simulink model "truck_mpc_8dof_2020a"  (R2020a)
settings: Solver=FixedStepAuto  StartTime=0.0  StopTime=40  FixedStep=0.001  RelTol=1e-3
libraries: neural x31, simulink x2, Solver_SF x1
(part 2 of 2)

== system truck_mpc_8dof_2020a/Feed-Forward Neural Network/Layer 4/Delays 1 ==
  "p{4}" : Inport  PortDimensions=6  SampleTime=0.0005
      mask Display: e = 0.06;c1 = [120 230 180]/255;c2 = ([120 230 180]+0)/(256+128);c3 = ([120 230 180]+128)/(256+128);patch([0 1 1 0],[0 0 1 1],c1);patch([0 1 1 1-e 1-e 0+e],[0 0 1 1-e 0+e 0+e],c2);patch([0 0 1 1-e 0+e 0+e],[0 1 1 1-e 1-e 0+e],c3);plot([0 1 1 0 0],[0 0 1 1 0]);
  mux : Mux  Inputs=1
      mask Display: e = 0.06;c1 = [120 150 230]/255;c2 = ([120 150 230]+0)/383;c3 = ([120 150 230]+128)/383;patch([0 1 1 0],[0 0 1 1],c1);patch([0 1 1 1-e 1-e 0+e],[0 0 1 1-e 0+e 0+e],c2);patch([0 0 1 1-e 0+e 0+e],[0 1 1 1-e 1-e 0+e],c3);plot([0 1 1 0 0],[0 0 1 1 0]);disp('Mux')
  "pd{4,3}" : Outport
      mask Display: e = 0.06;c1 = [120 230 180]/255;c2 = ([120 230 180]+0)/(256+128);c3 = ([120 230 180]+128)/(256+128);patch([0 1 1 0],[0 0 1 1],c1);patch([0 1 1 1-e 1-e 0+e],[0 0 1 1-e 0+e 0+e],c2);patch([0 0 1 1-e 0+e 0+e],[0 1 1 1-e 1-e 0+e],c3);plot([0 1 1 0 0],[0 0 1 1 0]);
  wires:
  "p{4}"/1 -> mux/1
  mux/1 -> "pd{4,3}"/1

== system truck_mpc_8dof_2020a/Feed-Forward Neural Network/Layer 4/LW{4,3} ==
  "ad{4,3}" : Inport  PortDimensions=6  SampleTime=0.0005
      mask Display: e = 0.06;c1 = [120 230 180]/255;c2 = ([120 230 180]+0)/(256+128);c3 = ([120 230 180]+128)/(256+128);patch([0 1 1 0],[0 0 1 1],c1);patch([0 1 1 1-e 1-e 0+e],[0 0 1 1-e 0+e 0+e],c2);patch([0 0 1 1-e 0+e 0+e],[0 1 1 1-e 1-e 0+e],c3);plot([0 1 1 0 0],[0 0 1 1 0]);
  "IW{4,3}(1,:)'" : Constant  Value=[1.0365086789271795719713509242865256965160369873046875;-0.07770699028544313102795371150932624004781246185302734375;-0.9449999401189803638345665603992529213428497314453125;0.1511782678576858440777641590102575719356536865234375;0.25449790728671828343721017517964355647563934326171875;-1.6818672952565700828841954717063345015048980712890625]
      mask Display: e = 0.06;c1 = [120 150 230]/255;c2 = ([120 150 230]+0)/383;c3 = ([120 150 230]+128)/383;patch([0 1 1 0],[0 0 1 1],c1);patch([0 1 1 1-e 1-e 0+e],[0 0 1 1-e 0+e 0+e],c2);patch([0 0 1 1-e 0+e 0+e],[0 1 1 1-e 1-e 0+e],c3);plot([0 1 1 0 0],[0 0 1 1 0]);disp('weights');
  Mux : Mux  Inputs=1
      mask Display: e = 0.06;c1 = [120 150 230]/255;c2 = ([120 150 230]+0)/383;c3 = ([120 150 230]+128)/383;patch([0 1 1 0],[0 0 1 1],c1);patch([0 1 1 1-e 1-e 0+e],[0 0 1 1-e 0+e 0+e],c2);patch([0 0 1 1-e 0+e 0+e],[0 1 1 1-e 1-e 0+e],c3);plot([0 1 1 0 0],[0 0 1 1 0]);disp('Mux');
  dotprod1 : neural/Weight Functions/dotprod
  "lz{4,3}" : Outport
      mask Display: e = 0.06;c1 = [120 230 180]/255;c2 = ([120 230 180]+0)/(256+128);c3 = ([120 230 180]+128)/(256+128);patch([0 1 1 0],[0 0 1 1],c1);patch([0 1 1 1-e 1-e 0+e],[0 0 1 1-e 0+e 0+e],c2);patch([0 0 1 1-e 0+e 0+e],[0 1 1 1-e 1-e 0+e],c3);plot([0 1 1 0 0],[0 0 1 1 0]);
  wires:
  "IW{4,3}(1,:)'"/1 -> dotprod1/1
  "ad{4,3}"/1 -> dotprod1/2
  dotprod1/1 -> Mux/1
  Mux/1 -> "lz{4,3}"/1

== matlab function truck_mpc_8dof_2020a/Speed PID controller/MATLAB Function1 ==
  data: u input; th output; b output
function [th, b]= fcn(u)

if u >= 0
    th=u;
    b=0;
elseif u<0
    th=0;
    b=u;
else
    th = 0;
    b = 0;
end

== matlab function truck_mpc_8dof_2020a/MPC Controller/MPC controller ==
  data: Xo input; steer output; Yo input; Yaw input; Yr input; V input; Vy input; Yaw_rate input; Yawr input
function steer = fcn(Xo, Yo, Yaw, Yr, V, Vy, Yaw_rate, Yawr)
x_k = [Yo-Yr;
       Yaw - Yawr;
       0;
       0]; %后两维可以编写一个误差获取的模块加在前面
N = 100;
%定义系统矩阵
q=[10,10,1,1];
Q = diag(q);
R = 1;
T = 0.001;

kf=140000;
km=120000;
kr=120000;
m=61000;
Iz=23665;
a=2.2;
b=2;
c=3.9;

if V <= 0.5
    V = 0.5;
end

tildeA = [1 V*T           T                              0                           ;
          0 1             0                              T                           ;
          0 0             1-T*(kf+km+kr)/(m*V)           -T*(a*kf-b*km-c*kr)/(m*V)-V*T    ;
          0 0             -T*(a*kf-b*km-c*kr)/(Iz*V)      1-T*(a*a*kf+b*b*km+c*c*kr)/(Iz*V)];

tildeB = [0;
          0;
          T*kf/m;
          T*a*kf/Iz];


n = size(tildeA,1);
p = size(tildeB,2);

Psi = zeros(N*n, n);
Theta = zeros(N*n,N*p);
tmp=eye(n);


for i = 1:N
    rows = (i-1)*n+(1:n);
    if i == 1
        Theta(rows, 1:p) = tmp*tildeB;
    else
        Theta(rows, :) = [tmp*tildeB, Theta(rows-n, 1:end-p)];
    end
    tmp = tildeA*tmp;
    Psi(rows,:) = tmp;
end

Q_bar = kron(eye(N),Q);
R_bar = kron(eye(N),R);

E = Theta'*Q_bar*Psi;
H = Theta'*Q_bar*Theta + R_bar;
error = Psi*x_k;
% print(size(error))
U_k = zeros(N*p, 1);
U_k = -H^-1*E*x_k;

steer = U_k(1:p,1);%1:p



% function steer = fcn(Xo, Yo ,Yaw, Yr, V, deltar)
% x_k = [Yo-Yr;
%         Yaw;
%         0];
% N = 100;
% %定义系统矩阵
% Q = [30 0 0;
%      0 20 0;
%      0 0 1];
% R = 0.5;
% T = 0.001;
% l=6.2;
% tildeA = [1 T*V*cos(deltar) 0;
%           0     1 T*V/(l*cos(deltar)^2);
%           0     0       -(1/0.2) + 1];
% 
% tildeB = [0;
%           0;
%           0.0005/0.2];
% 
% n = size(tildeA,1);
% p = size(tildeB,2);
% 
% Psi = zeros(N*n, n);
% Theta = zeros(N*n,N*p);
% tmp=eye(n);
% 
% 
% for i = 1:N
%     rows = (i-1)*n+(1:n);
%     if i == 1
%         Theta(rows, 1:p) = tmp*tildeB;
%     else
%         Theta(rows, :) = [tmp*tildeB, Theta(rows-n, 1:end-p)];
%     end
%     tmp = tildeA*tmp;
%     Psi(rows,:) = tmp;
% end
% 
% Q_bar = kron(eye(N),Q);
% R_bar = kron(eye(N),R);
% 
% E = Theta'*Q_bar*Psi;
% H = Theta'*Q_bar*Theta + R_bar;
% 
% U_k = zeros(N*p, 1);
% U_k = -H^-1*E*x_k;
% 
% steer = U_k(1,1);%1:p

== matlab function truck_mpc_8dof_2020a/Noise Generator ==
  data: steer input; esteer_sin_noise output; yaw input; speed input
function esteer_sin_noise = fcn(steer,yaw,speed)

esteer_sin_noise = 5*sin(0.11*steer)*sin(0.05*(yaw-51)) ...
*sin(1.18*speed)+0.15*sin(3.11*steer)*sin(1.05*(yaw-51));

== matlab function truck_mpc_8dof_2020a/MPC Controller/MATLAB Function1 ==
  data: x input; y output
function y = fcn(x)
r1=0.096*(x-60)-1.2;
r2=0.096*(x-120)-1.2;
dm1=25;
dm2=25;
dn1=3.6;
dn2=3.6;
y = dn1/2*(1+tanh(r1))-dn2/2*(1+tanh(r2));

== matlab function truck_mpc_8dof_2020a/MPC Controller/MATLAB Function2 ==
  data: x input; yaw output
function yaw = fcn(x)
r1=0.096*(x-60)-1.2;
r2=0.096*(x-120)-1.2;
dm1=25;
dm2=25;
dn1=3.6;
dn2=3.6;
yaw = atan(dn1*(1/cosh(r1))^2*(1.2/dm1)-dn2*(1/cosh(r2))^2*(1.2/dm2));

== matlab function truck_mpc_8dof_2020a/MPC Controller/MATLAB Function ==
  data: t input; u input; y output
function y = fcn(t, u)
if t <= 0.1
    u=0.000001;
end

if u >= 40
    u=40;
end

if u <= -40
    u=-40;
end

y = u;

== matlab function truck_mpc_8dof_2020a/数学模型 ==
  data: x input; u input; dotx output; V input
function dotx = fcn(x,u,V)

kf=140000;
km=120000;
kr=120000;
m=61000;
Iz=650000;
a=2.2;
b=2;
c=3.9;

if V <= 0.5
    V = 0.5;
end

A = [0 V           1                              0                           ;
     0 0           0                              1                           ;
     0 0           -(kf+km+kr)/(m*V)               -(a*kf-b*km-c*kr)/(m*V)-V    ;
     0 0           -(a*kf-b*km-c*kr)/(Iz*V)        -(a*a*kf+b*b*km+c*c*kr)/(Iz*V)];

B = [0;
     0;
     kf/m;
     a*kf/Iz];

dotx = A*x+B*u;

== matlab function truck_mpc_8dof_2020a/数学模型1 ==
  data: x input; u input; xdot output; V input
function xdot = fcn(x,u,V)
l=6.2;

xdot = [sin(x(2))*V;
        (tan(u)/l)*V];
